simulink model "IP_SwingUp_Design"  (R2024b)
settings: Solver=VariableStepAuto  StartTime=0.0  StopTime=15  FixedStep=0.01  RelTol=1e-3
values from neighbouring files (symbols this model uses):
  b = 0.00007892    (= 7.892e-05)    [Init_Setup_LQRArd.m]
  c = 0.63    [Init_Setup_LQRArd.m]
  g = 9.81    [Init_Setup_LQRArd.m]
  I = 0.0007176    [Init_Setup_LQRArd.m]
  kb = 0.031    [Init_Setup_LQRArd.m]
  KK = lqr(A_nom, B_nom, Q, R)    [Init_Setup_LQRArd.m]
  kt = 0.031    [Init_Setup_LQRArd.m]
  l = input('Longitud del péndulo (m): ')    [Init_Setup_LQRArd.m]
  M = 0.136    [Init_Setup_LQRArd.m]
  m = 0.1    [Init_Setup_LQRArd.m]
  M_c = 0.135    [Init_Setup_LQRArd.m]
  r = 0.006    [Init_Setup_LQRArd.m]
  Rm = 12.5    [Init_Setup_LQRArd.m]
undefined symbols (not defined in the file or in its folder): Er, n
libraries: vrlib x3, simulink x3
settings Model: Creator=jitendra  LastModifiedBy=lihao
settings SolverCC: AlgebraicLoopSolver=LineSearch
settings DataIOCC: ExternalInput=getinputstruct(op_trim1)  InitialState=getstatestruct(op_trim1)  ReturnWorkspaceOutputs=off
settings DebuggingCC: UnconnectedInputMsg=warning  UnconnectedOutputMsg=warning  UnconnectedLineMsg=warning  ArithmeticOperatorsInVariantConditions=warning
settings ModelReferenceCC: EnableRefExpFcnMdlSchedulingChecks=on
settings SFSimCC: SimUseLocalCustomCode=off  CustomCodeUndefinedFunction=UseInterfaceOnly
settings RTWCC: RTWUseLocalCustomCode=off  GPUComputeCapability=3.5

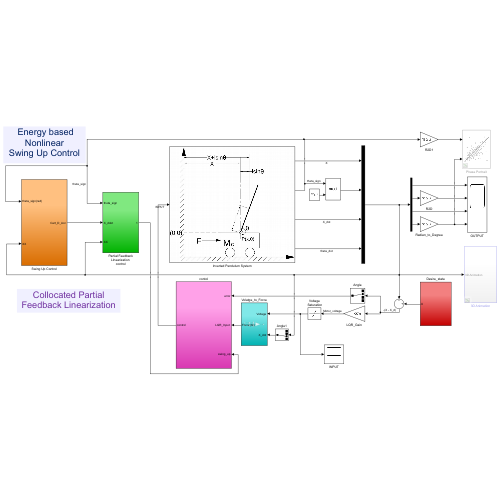
[thumbnail: Simulink's stored preview of the top-level diagram]
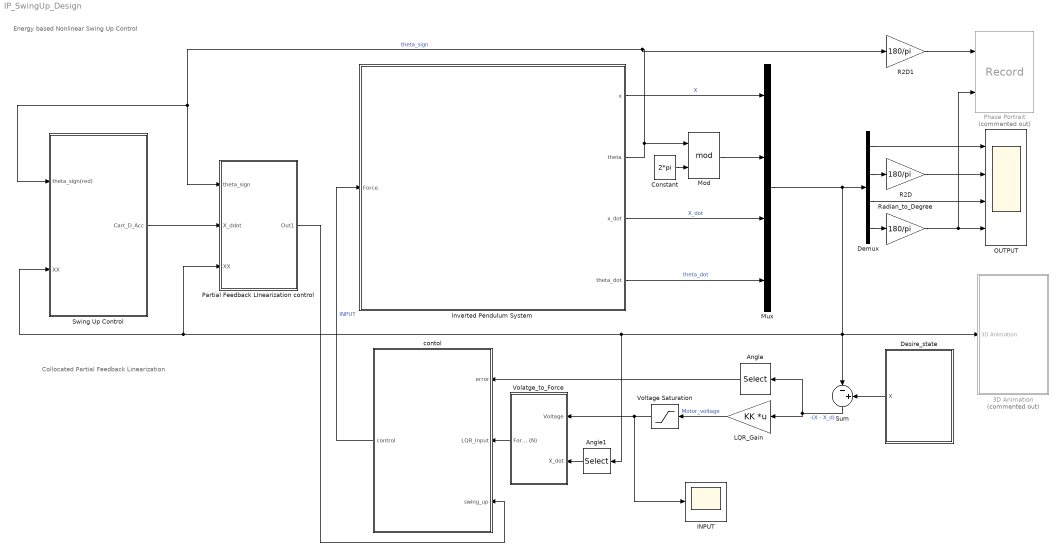
== system IP_SwingUp_Design ==
  note: Collocated Partial
      | Feedback Linearization
  note: Energy based
      | Nonlinear
      | Swing Up Control
  3D Animation : Subsystem  Commented=on
  Angle : Selector  InputPortWidth=4  IndexOptions=Index vector (dialog)  Indices=[2]  OutputSizes=1
  Angle1 : Selector  InputPortWidth=4  IndexOptions=Index vector (dialog)  Indices=[3]  OutputSizes=1
  Constant : Constant  Value=2*pi
  Demux : Demux
  Desire_state : Subsystem
  INPUT : Scope
  Inverted Pendulum System : Subsystem
      mask Display: image('ip_model.png');
  LQR_Gain : Gain  Gain=KK  Multiplication=Matrix(K*u)
  Mod : Math  Operator=mod  SignedPower=on
  Mux : Mux
  OUTPUT : Scope  NumInputPorts=4
  Partial Feedback LInearization control : Subsystem
  Phase Portrait : Record  Commented=on  FileSettingsInternal="{\"entries\":[{\"content\":{\"excelSettings\":{\"content\":{},\"type\":\"Streamout.ExcelSettings\"}},\"type\":\"Streamout.FileSettingStorage\",\"uuid\":\"\"}],\"packageUris\":[\"http:\\/\\/schema.mathworks.com\\/mf0\\/streamout_blocks\\/R2020a\"],\"version\":\"1.0\"}"  Layout=[1 1]  SignalsInternal="{\"entries\":[{\"content\":{\"signals\":[{\"content\":{\"blockPath\":[],\"dimensions\":[1],\"domain\":\"\",\"lineColor\":\"#a2142f\",\"plots\":[ 1 ],\"port\":1,\"signalID\":1,\"signalName\":\"XY Graph:1\"},\"type\":\"RecordBlkView.Signal\",\"uuid\":\"\"},{\"content\":{\"blockPath\":[],\"dimensions\":[1],\"domain\":\"\",\"lineColor\":\"#139fff\",\"plots\":[ 1 ],\"port\":2,\"signalID\":2,\"signalName\":\"XY Graph:2\"},\"type\":\"RecordBlkView.Signal\",\"uuid\":\"\"}]},\"type\":\"RecordBlkView.InputSignals\",\"uuid\":\"\"}],\"packageUris\":[\"http:\\/\\/schema.mathworks.com\\/mf0\\/streamout_blocks\\/R2020a\"],\"version\":\"1.0\"}"  VisualizationBindings="{\"xyplotplugin\":{\"info\":[{\"series\":[{\"bindingParametersList\":[{\"parameter\":\"X-Axis\",\"signalID\":1,\"signalName\":\"XY Graph:1\"},{\"parameter\":\"Y-Axis\",\"signalID\":2,\"signalName\":\"XY Graph:2\"}],\"seriesID\":0}],\"subplotID\":1}]}}"  CompatibilityTag=XY  st=-1
  R2D : Gain  Gain=180/pi
  R2D1 : Gain  Gain=180/pi
  Radian_to_Degree : Gain  Gain=180/pi
  Sum : Sum  Inputs=|-+
  Swing Up Control : Subsystem
  Volatge_to_Force : Subsystem
  Voltage Saturation : Saturate  UpperLimit=12  LowerLimit=-12
  contol : Subsystem
  wires:
  Inverted Pendulum System/3(x_dot) -> Mux/3  "X_dot"
  Inverted Pendulum System/1(x) -> Mux/1  "X"
  Inverted Pendulum System/4(theta_dot) -> Mux/4  "theta_dot"
  Mux/1 -> Demux/1, 3D Animation/1(3D Animation), Sum/1, Angle1/1, Swing Up Control/2(XX), Partial Feedback LInearization control/3(XX)
  Desire_state/1(X) -> Sum/2
  Sum/1 -> Angle/1, LQR_Gain/1  "-(X - X_d)"
  Demux/2 -> R2D/1
  Demux/1 -> OUTPUT/1
  Demux/3 -> OUTPUT/3
  Demux/4 -> Radian_to_Degree/1
  R2D/1 -> OUTPUT/2
  Swing Up Control/1(Cart_D_Acc) -> Partial Feedback LInearization control/2(X_ddot)
  Angle/1 -> contol/1(error)
  Constant/1 -> Mod/2
  Inverted Pendulum System/2(theta) -> R2D1/1, Partial Feedback LInearization control/1(theta_sign), Swing Up Control/1(theta_sign(red)), Mod/1  "theta_sign"
  Mod/1 -> Mux/2
  Partial Feedback LInearization control/1(Out1) -> contol/3(swing_up)
  Radian_to_Degree/1 -> Phase Portrait/2, OUTPUT/4
  R2D1/1 -> Phase Portrait/1
  contol/1(control) -> Inverted Pendulum System/1(Force)  "INPUT"
  LQR_Gain/1 -> Voltage Saturation/1  "Motor_voltage"
  Volatge_to_Force/1(Force (N)) -> contol/2("LQR_Input ")
  Angle1/1 -> Volatge_to_Force/2(X_dot)
  Voltage Saturation/1 -> INPUT/1, Volatge_to_Force/1(Voltage)

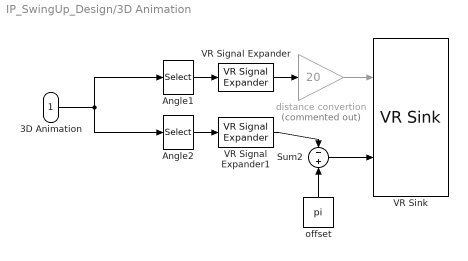
== system IP_SwingUp_Design/3D Animation ==
  3D Animation : Inport
  Angle1 : Selector  InputPortWidth=4  IndexOptions=Index vector (dialog)  Indices=[1]  OutputSizes=1
  Angle2 : Selector  InputPortWidth=4  IndexOptions=Index vector (dialog)  Indices=[2]  OutputSizes=1
  Sum2 : Sum  Inputs=-|+
  VR Signal Expander : vrlib/VR Signal Expander  outwidth=3  outidx=[1]
  VR Signal Expander1 : vrlib/VR Signal Expander  outwidth=4  outidx=[4]
  VR Sink : vrlib/VR Sink  InstantiateOnLoad=on  SampleTime=0.018  ViewEnable=on  RemoteChange=off  RemoteView=off  FieldsWritten=cart.translation.3.1.1.double#joint.rotation.4.1.1.double  WorldFileName=Inverted_pendulum12.wrl  AutoView=off  VideoDimensions=[]  AllowVariableSize=off  FigureProperties="{'Position', 'Name', 'Viewpoint', 'CameraBound', 'CameraDirection', 'CameraPosition', 'CameraUpVector', 'ZoomFactor', 'Antialiasing', 'Headlight', 'Lighting', 'Sound', 'StatusBar', 'Stereo3D', 'Stereo3DCameraOffset', 'Stereo3DHIT', 'ToolBar', 'Textures', 'Transparency', 'Triad', 'Wireframe', 'NavZones', 'NavMode', 'NavSpeed', 'CaptureFileFormat', 'CaptureFileName', 'Record2DCompressMethod', 'Record2DCompressQuality', 'Record2D', 'Record2DFileName', 'Record2DFPS', 'NavPanel'; [3.3060000000000002e+02   1.9979999999999995e+02   5.7600000000000000e+02   3.5000000000000000e+02], '', '', 'on', [0.0000000000000000e+00   0.0000000000000000e+00  -9.9999999999999989e-01], [0.0000000000000000e+00  -6.0000002384185791e-01   2.6254408740997309e+01], [0.0000000000000000e+00   1.0000000000000000e+00   0.0000000000000000e+00], [1.0000000000000000e+00], 'on', 'on', 'on', 'on', 'on', 'off', [1.0000000149011612e-01], [0.0000000000000000e+00], 'on', 'on', 'on', 'none', 'off', 'off', 'fly', 'normal', 'tif', '%f_anim_%n.tif', 'auto', [7.5000000000000000e+01], 'off', '%f_anim_%n.avi', 'auto', 'halfbar'}"
  distance convertion : Gain  Commented=on  Gain=20
  offset : Constant  Value=pi
  wires:
  VR Signal Expander/1 -> distance convertion/1
  3D Animation/1 -> Angle2/1, Angle1/1
  Angle1/1 -> VR Signal Expander/1
  Angle2/1 -> VR Signal Expander1/1
  offset/1 -> Sum2/2
  Sum2/1 -> VR Sink/2
  VR Signal Expander1/1 -> Sum2/1
  distance convertion/1 -> VR Sink/1

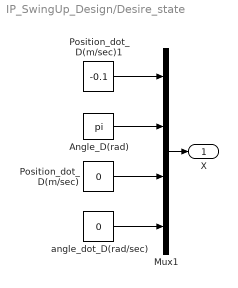
== system IP_SwingUp_Design/Desire_state ==
  Angle_D(rad) : Constant  Value=pi
  Mux1 : Mux
  Position_dot_D(m/sec) : Constant  Value=0
  Position_dot_D(m/sec)1 : Constant  Value=-0.1
  angle_dot_D(rad/sec) : Constant  Value=0
  X : Outport  VectorParamsAs1DForOutWhenUnconnected=off
  wires:
  Mux1/1 -> X/1
  Position_dot_D(m/sec)/1 -> Mux1/3
  angle_dot_D(rad/sec)/1 -> Mux1/4
  Angle_D(rad)/1 -> Mux1/2
  Position_dot_D(m/sec)1/1 -> Mux1/1

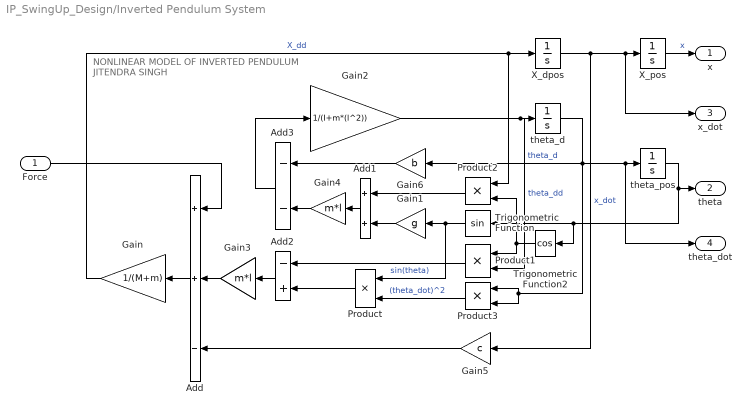
== system IP_SwingUp_Design/Inverted Pendulum System ==
  note: NONLINEAR MODEL OF
      | INVERTED PENDULUM
      | JITENDRA SINGH
  Force : Inport
  Add : Sum  Inputs=++-
  Add1 : Sum
  Add2 : Sum  Inputs=-+
  Add3 : Sum  Inputs=--
  Gain : Gain  Gain=1/(M+m)
  Gain1 : Gain  Gain=g
  Gain2 : Gain  Gain=1/(I+m*(l^2))
  Gain3 : Gain  Gain=m*l
  Gain4 : Gain  Gain=m*l
  Gain5 : Gain  Gain=c
  Gain6 : Gain  Gain=b
  Product{,1..3} (4 alike) : Product
  Trigonometric Function : Trigonometry
  Trigonometric Function2 : Trigonometry  Operator=cos
  X_dpos : Integrator
  X_pos : Integrator
  theta_d : Integrator
  theta_pos : Integrator  InitialCondition=1*(pi/180)
  x : Outport  VectorParamsAs1DForOutWhenUnconnected=off
  theta : Outport  Port=2  VectorParamsAs1DForOutWhenUnconnected=off
  x_dot : Outport  Port=3  VectorParamsAs1DForOutWhenUnconnected=off
  theta_dot : Outport  Port=4  VectorParamsAs1DForOutWhenUnconnected=off
  wires:
  Gain5/1 -> Add/3
  Add2/1 -> Gain3/1
  Add3/1 -> Gain2/1
  Trigonometric Function2/1 -> Product2/2, Product1/1
  Trigonometric Function/1 -> Product/1, Gain1/1  "sin(theta)"
  Gain3/1 -> Add/2
  theta_d/1 -> Product3/2, Product3/1, Gain6/1, theta_dot/1, theta_pos/1  "theta_d"
  Product2/1 -> Add1/1
  Product/1 -> Add2/2
  Gain4/1 -> Add3/2
  Product3/1 -> Product/2  "(theta_dot)^2"
  X_pos/1 -> x/1  "x"
  Product1/1 -> Add2/1
  Gain/1 -> X_dpos/1, Product2/1  "X_dd"
  Add/1 -> Gain/1
  Gain2/1 -> Product1/2, theta_d/1  "theta_dd"
  Gain6/1 -> Add3/1
  theta_pos/1 -> Trigonometric Function2/1, Trigonometric Function/1, theta/1
  Force/1 -> Add/1
  Gain1/1 -> Add1/2
  X_dpos/1 -> x_dot/1, X_pos/1, Gain5/1  "x_dot"
  Add1/1 -> Gain4/1

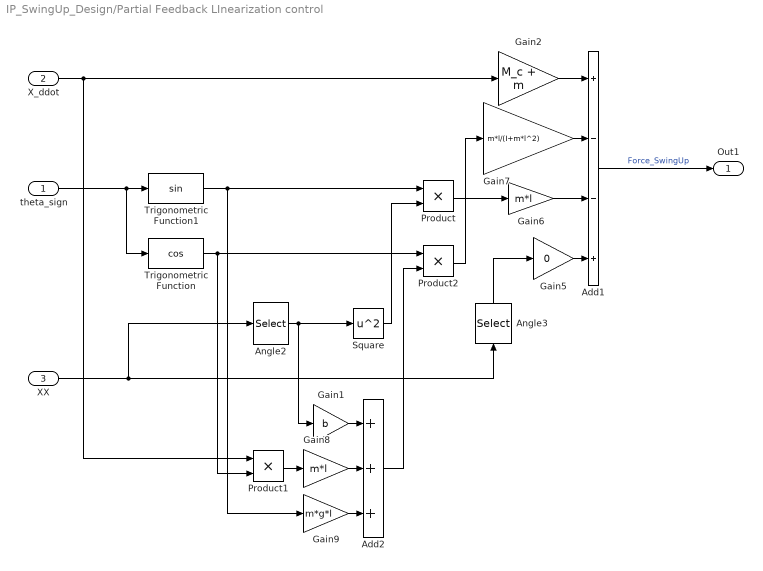
== system IP_SwingUp_Design/Partial Feedback LInearization control ==
  theta_sign : Inport
  X_ddot : Inport  Port=2
  XX : Inport  Port=3
  Add1 : Sum  Inputs=+--+
  Add2 : Sum  Inputs=+++
  Angle2 : Selector  InputPortWidth=4  IndexOptions=Index vector (dialog)  Indices=[4]  OutputSizes=1
  Angle3 : Selector  InputPortWidth=4  IndexOptions=Index vector (dialog)  Indices=[3]  OutputSizes=1
  Gain1 : Gain  Gain=b
  Gain2 : Gain  Gain=M_c + m
  Gain5 : Gain  Gain=0
  Gain6 : Gain  Gain=m*l
  Gain7 : Gain  Gain=m*l/(I+m*l^2)
  Gain8 : Gain  Gain=m*l
  Gain9 : Gain  Gain=m*g*l
  Product : Product
  Product1 : Product
  Product2 : Product
  Square : Math  Operator=square  SignedPower=on  RndMeth=Zero
  Trigonometric Function : Trigonometry  Operator=cos
  Trigonometric Function1 : Trigonometry
  Out1 : Outport  VectorParamsAs1DForOutWhenUnconnected=off
  wires:
  Angle3/1 -> Gain5/1
  X_ddot/1 -> Gain2/1, Product1/1
  Gain2/1 -> Add1/1
  Add1/1 -> Out1/1  "Force_SwingUp"
  Gain5/1 -> Add1/4
  Gain7/1 -> Add1/2
  theta_sign/1 -> Trigonometric Function/1, Trigonometric Function1/1
  XX/1 -> Angle3/1, Angle2/1
  Angle2/1 -> Square/1, Gain1/1
  Product/1 -> Gain6/1
  Trigonometric Function1/1 -> Product/1, Gain9/1
  Square/1 -> Product/2
  Gain6/1 -> Add1/3
  Gain1/1 -> Add2/1
  Product1/1 -> Gain8/1
  Trigonometric Function/1 -> Product2/1, Product1/2
  Gain8/1 -> Add2/2
  Gain9/1 -> Add2/3
  Add2/1 -> Product2/2
  Product2/1 -> Gain7/1

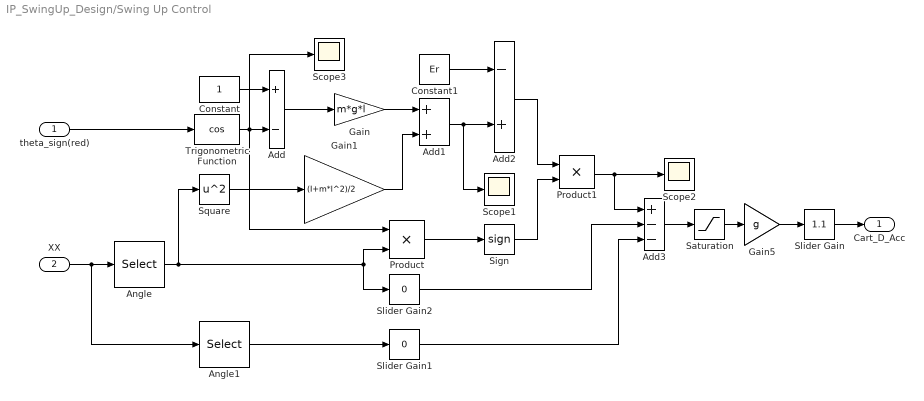
== system IP_SwingUp_Design/Swing Up Control ==
  theta_sign(red) : Inport
  XX : Inport  Port=2
  Add : Sum  Inputs=+-
  Add1 : Sum
  Add2 : Sum  Inputs=-+
  Add3 : Sum  Inputs=+--
  Angle : Selector  InputPortWidth=4  IndexOptions=Index vector (dialog)  Indices=[4]  OutputSizes=1
  Angle1 : Selector  InputPortWidth=4  IndexOptions=Index vector (dialog)  Indices=[1]  OutputSizes=1
  Constant : Constant
  Constant1 : Constant  Value=Er
  Gain : Gain  Gain=m*g*l
  Gain1 : Gain  Gain=(I+m*l^2)/2
  Gain5 : Gain  Gain=g
  Product : Product
  Product1 : Product
  Saturation : Saturate  UpperLimit=n*g  LowerLimit=-n*g
  Scope1 : Scope
  Scope2 : Scope
  Scope3 : Scope
  Sign : Signum
  Slider Gain : simulink/Math Operations/Slider Gain  gain=1.1  low=0  high=30
  Slider Gain1 : simulink/Math Operations/Slider Gain  gain=0  low=0  high=5
  Slider Gain2 : simulink/Math Operations/Slider Gain  gain=0  low=0  high=5
  Square : Math  Operator=square  SignedPower=on  RndMeth=Zero
  Trigonometric Function : Trigonometry  Operator=cos
  Cart_D_Acc : Outport  VectorParamsAs1DForOutWhenUnconnected=off
  wires:
  Constant/1 -> Add/1
  Add/1 -> Gain/1
  Trigonometric Function/1 -> Scope3/1, Product/1, Add/2
  Square/1 -> Gain1/1
  XX/1 -> Angle1/1, Angle/1
  Gain/1 -> Add1/1
  Gain1/1 -> Add1/2
  Product/1 -> Sign/1
  Add1/1 -> Scope1/1, Add2/2
  Add2/1 -> Product1/1
  Sign/1 -> Product1/2
  Product1/1 -> Scope2/1, Add3/1
  Saturation/1 -> Gain5/1
  Slider Gain/1 -> Cart_D_Acc/1
  Gain5/1 -> Slider Gain/1
  theta_sign(red)/1 -> Trigonometric Function/1
  Constant1/1 -> Add2/1
  Angle/1 -> Slider Gain2/1, Product/2, Square/1
  Angle1/1 -> Slider Gain1/1
  Slider Gain2/1 -> Add3/2
  Slider Gain1/1 -> Add3/3
  Add3/1 -> Saturation/1

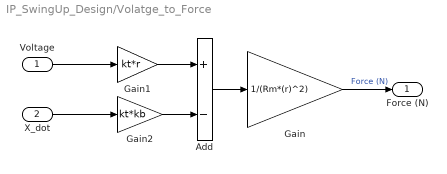
== system IP_SwingUp_Design/Volatge_to_Force ==
  Voltage : Inport
  X_dot : Inport  Port=2
  Add : Sum  Inputs=+-
  Gain : Gain  Gain=1/(Rm*(r)^2)
  Gain1 : Gain  Gain=kt*r
  Gain2 : Gain  Gain=kt*kb
  Force (N) : Outport  VectorParamsAs1DForOutWhenUnconnected=off
  wires:
  Gain1/1 -> Add/1
  Gain2/1 -> Add/2
  Voltage/1 -> Gain1/1
  Gain/1 -> Force (N)/1  "Force (N)"
  X_dot/1 -> Gain2/1
  Add/1 -> Gain/1

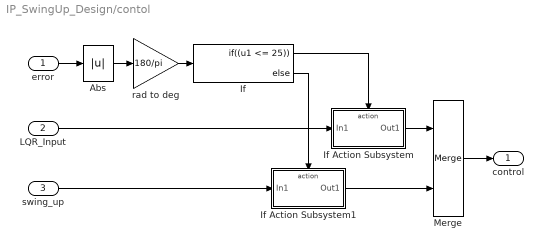
== system IP_SwingUp_Design/contol ==
  error : Inport
  "LQR_Input " : Inport  Port=2
  swing_up : Inport  Port=3
  Abs : Abs  SaturateOnIntegerOverflow=off
  If : If  IfExpression=(u1 <= 25)
  If Action Subsystem : Subsystem  TreatAsAtomicUnit=on
  If Action Subsystem1 : Subsystem  TreatAsAtomicUnit=on
  Merge : Merge
  rad to deg : Gain  Gain=180/pi
  control : Outport  VectorParamsAs1DForOutWhenUnconnected=off
  wires:
  Merge/1 -> control/1
  If/1 -> If Action Subsystem/Action
  If/2 -> If Action Subsystem1/Action
  swing_up/1 -> If Action Subsystem1/1(In1)
  If Action Subsystem1/1(Out1) -> Merge/2
  error/1 -> Abs/1
  Abs/1 -> rad to deg/1
  rad to deg/1 -> If/1
  If Action Subsystem/1(Out1) -> Merge/1
  "LQR_Input "/1 -> If Action Subsystem/1(In1)

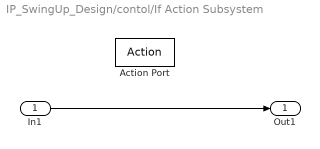
== system IP_SwingUp_Design/contol/If Action Subsystem ==
  In1 : Inport
  Action Port : ActionPort  ActionPortLabel=if((u1 <= 25))
  Out1 : Outport  VectorParamsAs1DForOutWhenUnconnected=off
  wires:
  In1/1 -> Out1/1

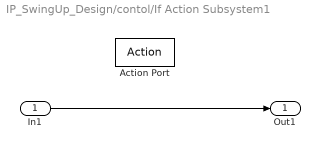
== system IP_SwingUp_Design/contol/If Action Subsystem1 ==
  In1 : Inport
  Action Port : ActionPort  ActionPortLabel=else
  Out1 : Outport  VectorParamsAs1DForOutWhenUnconnected=off
  wires:
  In1/1 -> Out1/1
